simulink model "fuzzy_impedence_control_1"  (R2018b)
settings: Solver=VariableStepAuto  StartTime=0.0  StopTime=100  RelTol=1e-3
libraries: fuzblock x1
settings Model: Creator=vojislav  LastModifiedBy=Nick

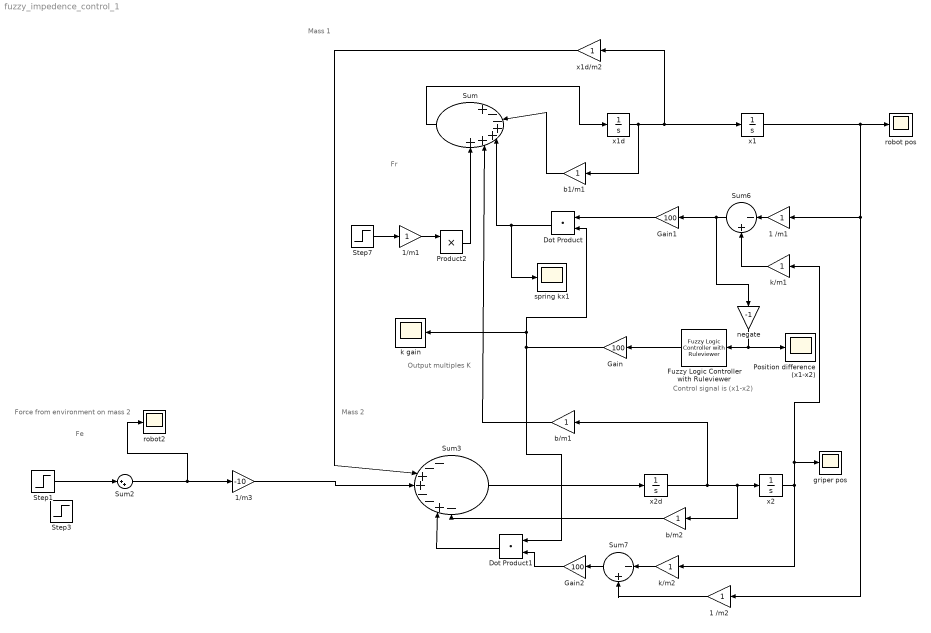
== system fuzzy_impedence_control_1 ==
  note: Fr
  note: Fe
  note: Force from environment
      | on mass 2
  note: Mass 1
  note: Mass 2
  note: Control signal is (x1-x2)
  note: Output multiples K
  1 /m1 : Gain
  1 /m2 : Gain
  1/m1 : Gain
  1/m3 : Gain  Gain=-10
  Dot Product : DotProduct  InputSameDT=on  OutDataTypeStr=Inherit: Inherit via internal rule
  Dot Product1 : DotProduct  InputSameDT=on  OutDataTypeStr=Inherit: Inherit via internal rule
  Fuzzy Logic Controller with Ruleviewer : fuzblock/Fuzzy Logic  Controller  with Ruleviewer  fismatrix=fuzzyKerror  Ts=2
  Gain : Gain  Gain=100
  Gain1 : Gain  Gain=100
  Gain2 : Gain  Gain=100
  Position difference (x1-x2) : Scope
  Product2 : Product
  Step1 : Step  Time=0  SampleTime=0
  Step3 : Step  Time=4  After=-1  SampleTime=0
  Step7 : Step  Time=0  Before=1  After=0  SampleTime=0
  Sum : Sum  Inputs=|+--++++
  Sum2 : Sum  Inputs=|++
  Sum3 : Sum  Inputs=|--++--+-
  Sum6 : Sum  Inputs=|-+
  Sum7 : Sum  Inputs=|-+
  b/m1 : Gain
  b/m2 : Gain
  b1/m1 : Gain
  griper pos : Scope
  "k gain " : Scope
  k/m1 : Gain
  k/m2 : Gain
  negate : Gain  Gain=-1
  robot pos : Scope
  robot2 : Scope
  spring kx1 : Scope
  x1 : Integrator
  x1d : Integrator
  x1d/m2 : Gain
  x2 : Integrator
  x2d : Integrator
  wires:
  Sum/1 -> x1d/1
  x1d/1 -> x1/1, x1d/m2/1, b1/m1/1
  Sum3/1 -> x2d/1
  x2d/1 -> b/m1/1, x2/1, b/m2/1
  b1/m1/1 -> Sum/3
  x1/1 -> 1 /m1/1, 1 /m2/1, robot pos/1
  Step1/1 -> Sum2/1
  Sum2/1 -> 1/m3/1, robot2/1
  1/m3/1 -> Sum3/4
  x2/1 -> k/m1/1, griper pos/1, k/m2/1
  1 /m1/1 -> Sum6/1
  k/m1/1 -> Sum6/2
  Sum6/1 -> Gain1/1, negate/1
  k/m2/1 -> Sum7/1
  Sum7/1 -> Gain2/1
  Step7/1 -> 1/m1/1
  Dot Product/1 -> spring kx1/1, Sum/5
  b/m1/1 -> Sum/6
  1 /m2/1 -> Sum7/2
  Gain/1 -> Dot Product1/1, Dot Product/2, "k gain "/1
  Gain1/1 -> Dot Product/1
  Gain2/1 -> Dot Product1/2
  1/m1/1 -> Product2/1
  Product2/1 -> Sum/7
  negate/1 -> Fuzzy Logic Controller with Ruleviewer/1, Position difference (x1-x2)/1
  b/m2/1 -> Sum3/8
  Dot Product1/1 -> Sum3/7
  x1d/m2/1 -> Sum3/3
  Fuzzy Logic Controller with Ruleviewer/1 -> Gain/1
